simulink model "Clutch_Pedal"  (R2020b)
settings: Solver=VariableStepAuto  StartTime=0.0  StopTime=10.0  RelTol=1e-3
values from neighbouring files (symbols this model uses):
  be = 2.0    [clutch_parameters.sldd]
  bv = 1.0    [clutch_parameters.sldd]
  Ie = 1.0    [clutch_parameters.sldd]
  Iv = 5.0    [clutch_parameters.sldd]
  R = 1.0    [clutch_parameters.sldd]
  uk = 1.0    [clutch_parameters.sldd]
  us = 1.5    [clutch_parameters.sldd]
undefined symbols (not defined in the file or in its folder): sigbuilder_block
settings Model: DataDictionary=clutch_parameters.sldd  Creator=shivanshu shukla  LastModifiedBy=shivanshu shukla

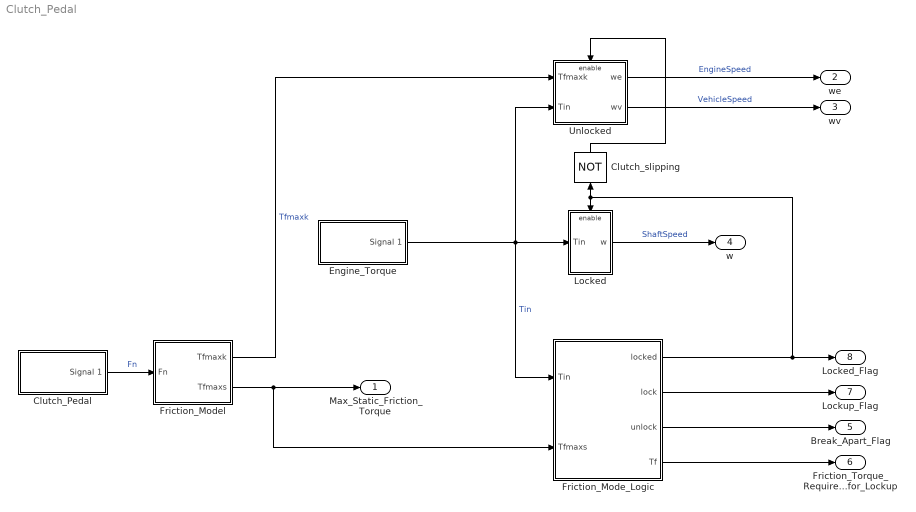
== system Clutch_Pedal ==
  Clutch_Pedal : Subsystem  Tag=STV Subsys  LoadFcn=sigbuilder_block('load');  StartFcn=sigbuilder_block('start');  StopFcn=sigbuilder_block('stop');  ClipboardFcn=sigbuilder_block('clipboard');  mask(Sigbuilder block){tuvar=[0:10]}
      mask help: Simulink:masks:SigbuilderBlock_MD
      mask init:
      | if ~strcmp(get_param(bdroot(gcbh),'SimulationStatus'),'stopped') tuvar = sigbuilder_block('maskInit'); end
      settings: CopyFcn=sigbuilder_block('copy');  DeleteFcn=sigbuilder_block('delete');  ModelCloseFcn=sigbuilder_block('modelClose');  PreSaveFcn=sigbuilder_block('preSave');  PauseFcn=sigbuilder_block('pause');  ContinueFcn=sigbuilder_block('continue');  NameChangeFcn=sigbuilder_block('namechange');  OpenFcn=sigbuilder_block('open',[437.6 153 550.4 359.25 ]);  CloseFcn=sigbuilder_block('close');
      mask Display: plot(0, 0, 100, 100,[2, 2, 32, 32, 2], [68, 8, 8, 68, 68],[32, 2], [38, 38], [32, 19, 2],[53, 60, 44], [32, 17, 17, 2],[16, 16, 31, 31]);txt = getActiveGroup(gcbh);text(2, 100, txt,'verticalAlignment', 'top');
  Clutch_slipping : Logic  Operator=NOT  IconShape=distinctive  AllPortsSameDT=off  OutDataTypeStr=boolean
  Engine_Torque : Subsystem  Tag=STV Subsys  LoadFcn=sigbuilder_block('load');  StartFcn=sigbuilder_block('start');  StopFcn=sigbuilder_block('stop');  ClipboardFcn=sigbuilder_block('clipboard');  mask(Sigbuilder block){tuvar=[0:10]}
      mask help: Simulink:masks:SigbuilderBlock_MD
      mask init:
      | if ~strcmp(get_param(bdroot(gcbh),'SimulationStatus'),'stopped') tuvar = sigbuilder_block('maskInit'); end
      settings: CopyFcn=sigbuilder_block('copy');  DeleteFcn=sigbuilder_block('delete');  ModelCloseFcn=sigbuilder_block('modelClose');  PreSaveFcn=sigbuilder_block('preSave');  PauseFcn=sigbuilder_block('pause');  ContinueFcn=sigbuilder_block('continue');  NameChangeFcn=sigbuilder_block('namechange');  OpenFcn=sigbuilder_block('open',[437.6 153 550.4 359.25 ]);  CloseFcn=sigbuilder_block('close');
      mask Display: plot(0, 0, 100, 100,[2, 2, 32, 32, 2], [68, 8, 8, 68, 68],[32, 2], [38, 38], [32, 19, 2],[53, 60, 44], [32, 17, 17, 2],[16, 16, 31, 31]);txt = getActiveGroup(gcbh);text(2, 100, txt,'verticalAlignment', 'top');
  Friction_Mode_Logic : Subsystem
  Friction_Model : Subsystem
  Locked : Subsystem
  Unlocked : Subsystem
  Max_Static_Friction_Torque : Outport
  we : Outport  Port=2
  wv : Outport  Port=3
  w : Outport  Port=4
  Break_Apart_Flag : Outport  Port=5
  Friction_Torque_Required_for_Lockup : Outport  Port=6
  Lockup_Flag : Outport  Port=7
  Locked_Flag : Outport  Port=8
  wires:
  Clutch_slipping/1 -> Unlocked/Enable
  Friction_Mode_Logic/1(locked) -> Locked_Flag/1, Clutch_slipping/1, Locked/Enable
  Friction_Model/1(Tfmaxk) -> Unlocked/1(Tfmaxk)  "Tfmaxk"
  Friction_Model/2(Tfmaxs) -> Max_Static_Friction_Torque/1, Friction_Mode_Logic/2(Tfmaxs)
  Engine_Torque/1(Signal 1) -> Friction_Mode_Logic/1(Tin), Locked/1(Tin), Unlocked/2(Tin)  "Tin"
  Clutch_Pedal/1(Signal 1) -> Friction_Model/1(Fn)  "Fn"
  Unlocked/1(we) -> we/1  "EngineSpeed"
  Unlocked/2(wv) -> wv/1  "VehicleSpeed"
  Locked/1(w) -> w/1  "ShaftSpeed"
  Friction_Mode_Logic/2(lock) -> Lockup_Flag/1
  Friction_Mode_Logic/3(unlock) -> Break_Apart_Flag/1
  Friction_Mode_Logic/4(Tf) -> Friction_Torque_Required_for_Lockup/1

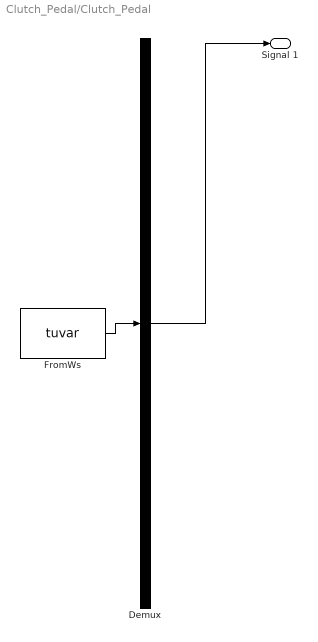
== system Clutch_Pedal/Clutch_Pedal ==
  Demux : Demux  Tag=STV Demux  Outputs=1
      settings: DisplayOption=none
  FromWs : FromWorkspace  Tag=STV FromWs  VariableName=tuvar
      SigBuilderData=|
      | common.afterFinalStr = 'Extrapolate'
      | common.sampleTime = 0
      | dataSet.timeRange = [0 10]
      | dataSet.name = 'Group 1'
      | sbobj.Groups.Name = 'Group 1'
      | sbobj.Groups.Signals.Name = 'Signal 1'
      | sbobj.Groups.Signals.XData = [0 1.98 3.96 4.98 6 7 7 10]
      | sbobj.Groups.Signals.YData = [0 1.6 1.6 1.6 0.83 -0.01 0 0]
  Signal 1 : Outport  Tag=STV Outport
  wires:
  Demux/1 -> Signal 1/1
  FromWs/1 -> Demux/1

== system Clutch_Pedal/Engine_Torque ==
  Demux : Demux  Tag=STV Demux  Outputs=1
      settings: DisplayOption=none
  FromWs : FromWorkspace  Tag=STV FromWs  VariableName=tuvar
      SigBuilderData=|
      | common.afterFinalStr = 'Extrapolate'
      | common.sampleTime = 0
      | dataSet.timeRange = [0 10]
      | dataSet.name = 'Group 1'
      | sbobj.Groups.Name = 'Group 1'
      | sbobj.Groups.Signals.Name = 'Signal 1'
      | sbobj.Groups.Signals.XData = [0 4 5.02 6 7 10]
      | sbobj.Groups.Signals.YData = [1.98 1.99 2 0.02 0 0]
  Signal 1 : Outport  Tag=STV Outport
  wires:
  Demux/1 -> Signal 1/1
  FromWs/1 -> Demux/1

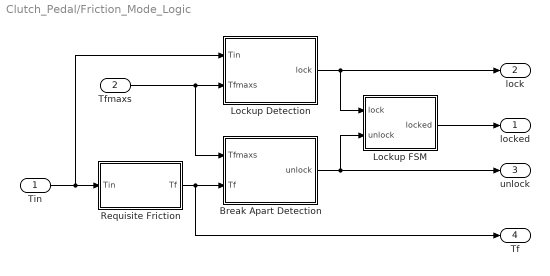
== system Clutch_Pedal/Friction_Mode_Logic ==
  Tin : Inport
  Tfmaxs : Inport  Port=2
  Break Apart Detection : Subsystem
  Lockup Detection : Subsystem
  Lockup FSM : Subsystem
  Requisite Friction : Subsystem
  locked : Outport  InitialOutput=0  VectorParamsAs1DForOutWhenUnconnected=off
  lock : Outport  Port=2  InitialOutput=0  VectorParamsAs1DForOutWhenUnconnected=off
  unlock : Outport  Port=3  InitialOutput=0  VectorParamsAs1DForOutWhenUnconnected=off
  Tf : Outport  Port=4  InitialOutput=0  VectorParamsAs1DForOutWhenUnconnected=off
  wires:
  Requisite Friction/1(Tf) -> Tf/1, Break Apart Detection/2(Tf)
  Break Apart Detection/1(unlock) -> unlock/1, Lockup FSM/2(unlock)
  Lockup FSM/1(locked) -> locked/1
  Tin/1 -> Lockup Detection/1(Tin), Requisite Friction/1(Tin)
  Lockup Detection/1(lock) -> lock/1, Lockup FSM/1(lock)
  Tfmaxs/1 -> Lockup Detection/2(Tfmaxs), Break Apart Detection/1(Tfmaxs)

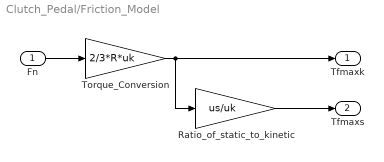
== system Clutch_Pedal/Friction_Model ==
  Fn : Inport
  Ratio_of_static_to_kinetic : Gain  Gain=us/uk  SaturateOnIntegerOverflow=on  OutDataTypeStr=Inherit: Same as input  ParamDataTypeStr=Inherit: Same as input
  Torque_Conversion : Gain  Gain=2/3*R*uk  SaturateOnIntegerOverflow=on  OutDataTypeStr=Inherit: Same as input  ParamDataTypeStr=Inherit: Same as input
  Tfmaxk : Outport  InitialOutput=0  VectorParamsAs1DForOutWhenUnconnected=off
  Tfmaxs : Outport  Port=2  InitialOutput=0  VectorParamsAs1DForOutWhenUnconnected=off
  wires:
  Torque_Conversion/1 -> Tfmaxk/1, Ratio_of_static_to_kinetic/1
  Ratio_of_static_to_kinetic/1 -> Tfmaxs/1
  Fn/1 -> Torque_Conversion/1

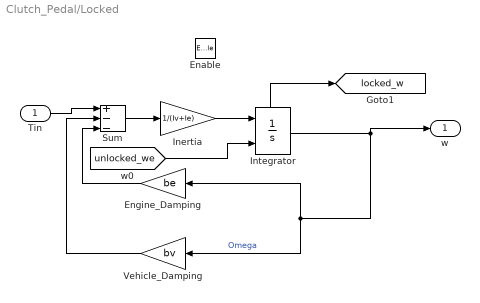
== system Clutch_Pedal/Locked ==
  Tin : Inport
  Enable : EnablePort  StatesWhenEnabling=reset
  Engine_Damping : Gain  Gain=be  SaturateOnIntegerOverflow=on  OutDataTypeStr=Inherit: Same as input  ParamDataTypeStr=Inherit: Same as input
  Inertia : Gain  Gain=1/(Iv+Ie)  SaturateOnIntegerOverflow=on  OutDataTypeStr=Inherit: Same as input  ParamDataTypeStr=Inherit: Same as input
  Integrator : Integrator  InitialConditionSource=external  ShowStatePort=on
  Sum : Sum  Inputs=+--  InputSameDT=on  SaturateOnIntegerOverflow=on  OutDataTypeStr=Inherit: Same as first input
  Vehicle_Damping : Gain  Gain=bv  SaturateOnIntegerOverflow=on  OutDataTypeStr=Inherit: Same as input  ParamDataTypeStr=Inherit: Same as input
  w : Outport  InitialOutput=0  VectorParamsAs1DForOutWhenUnconnected=off
  tag scope: locked_w=global
  wires:
  Engine_Damping/1 -> Sum/3
  Integrator/1 -> w/1, Engine_Damping/1, Vehicle_Damping/1  "Omega"
  Vehicle_Damping/1 -> Sum/2
  Tin/1 -> Sum/1
  Inertia/1 -> Integrator/1
  Sum/1 -> Inertia/1
  [unlocked_we] -> Integrator/2
  Integrator/State -> [locked_w]

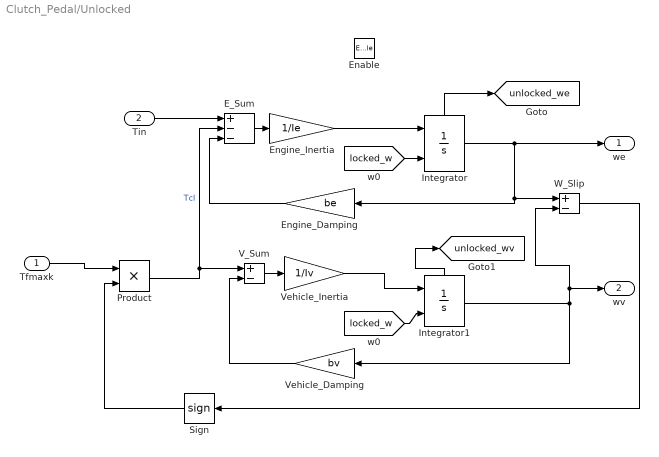
== system Clutch_Pedal/Unlocked ==
  Tfmaxk : Inport
  Tin : Inport  Port=2
  Enable : EnablePort
  E_Sum : Sum  Inputs=+--  InputSameDT=on  SaturateOnIntegerOverflow=on  OutDataTypeStr=Inherit: Same as first input
  Engine_Damping : Gain  Gain=be  SaturateOnIntegerOverflow=on  OutDataTypeStr=Inherit: Same as input  ParamDataTypeStr=Inherit: Same as input
  Engine_Inertia : Gain  Gain=1/Ie  SaturateOnIntegerOverflow=on  OutDataTypeStr=Inherit: Same as input  ParamDataTypeStr=Inherit: Same as input
  Integrator : Integrator  InitialConditionSource=external  ShowStatePort=on
  Integrator1 : Integrator  InitialConditionSource=external  ShowStatePort=on
  Product : Product
  Sign : Signum
  V_Sum : Sum  Inputs=+-  InputSameDT=on  SaturateOnIntegerOverflow=on  OutDataTypeStr=Inherit: Same as first input
  Vehicle_Damping : Gain  Gain=bv  SaturateOnIntegerOverflow=on  OutDataTypeStr=Inherit: Same as input  ParamDataTypeStr=Inherit: Same as input
  Vehicle_Inertia : Gain  Gain=1/Iv  SaturateOnIntegerOverflow=on  OutDataTypeStr=Inherit: Same as input  ParamDataTypeStr=Inherit: Same as input
  W_Slip : Sum  Inputs=+-  InputSameDT=on  SaturateOnIntegerOverflow=on  OutDataTypeStr=Inherit: Same as first input
  we : Outport  InitialOutput=0  VectorParamsAs1DForOutWhenUnconnected=off
  wv : Outport  Port=2  InitialOutput=0  VectorParamsAs1DForOutWhenUnconnected=off
  tag scope: unlocked_we=global, unlocked_wv=global
  wires:
  Vehicle_Damping/1 -> V_Sum/2
  Product/1 -> V_Sum/1, E_Sum/2  "Tcl"
  Vehicle_Inertia/1 -> Integrator1/1
  Tfmaxk/1 -> Product/1
  Integrator/1 -> we/1, Engine_Damping/1, W_Slip/1
  V_Sum/1 -> Vehicle_Inertia/1
  Engine_Damping/1 -> E_Sum/3
  Tin/1 -> E_Sum/1
  Integrator1/1 -> W_Slip/2, wv/1, Vehicle_Damping/1
  W_Slip/1 -> Sign/1
  E_Sum/1 -> Engine_Inertia/1
  Engine_Inertia/1 -> Integrator/1
  Sign/1 -> Product/2
  [locked_w] -> Integrator/2
  Integrator/State -> [unlocked_we]
  Integrator1/State -> [unlocked_wv]
  [locked_w] -> Integrator1/2

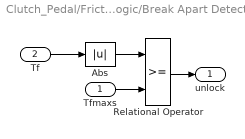
== system Clutch_Pedal/Friction_Mode_Logic/Break Apart Detection ==
  Tfmaxs : Inport
  Tf : Inport  Port=2
  Abs : Abs  SaturateOnIntegerOverflow=on
  Relational Operator : RelationalOperator  OutDataTypeStr=boolean  RndMeth=Nearest  InputSameDT=on
  unlock : Outport  InitialOutput=0  VectorParamsAs1DForOutWhenUnconnected=off
  wires:
  Tf/1 -> Abs/1
  Relational Operator/1 -> unlock/1
  Abs/1 -> Relational Operator/1
  Tfmaxs/1 -> Relational Operator/2

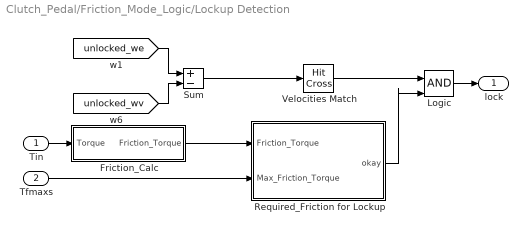
== system Clutch_Pedal/Friction_Mode_Logic/Lockup Detection ==
  Tin : Inport
  Tfmaxs : Inport  Port=2
  Friction_Calc : Subsystem
  Logic : Logic  IconShape=distinctive  OutDataTypeStr=boolean
  Required_Friction for Lockup : Subsystem
  Sum : Sum  Inputs=+-  InputSameDT=on  SaturateOnIntegerOverflow=on  OutDataTypeStr=Inherit: Same as first input
  Velocities Match : HitCross
  lock : Outport  InitialOutput=0  VectorParamsAs1DForOutWhenUnconnected=off
  wires:
  Tfmaxs/1 -> Required_Friction for Lockup/2(Max_Friction_Torque)
  Velocities Match/1 -> Logic/1
  Logic/1 -> lock/1
  Required_Friction for Lockup/1(okay) -> Logic/2
  [unlocked_we] -> Sum/1
  [unlocked_wv] -> Sum/2
  Sum/1 -> Velocities Match/1
  Tin/1 -> Friction_Calc/1(Torque)
  Friction_Calc/1(Friction_Torque) -> Required_Friction for Lockup/1(Friction_Torque)

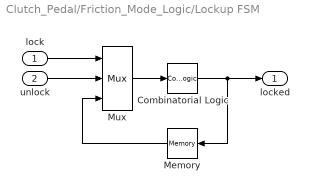
== system Clutch_Pedal/Friction_Mode_Logic/Lockup FSM ==
  lock : Inport
  unlock : Inport  Port=2
  Combinatorial Logic : CombinatorialLogic  TruthTable=[0;1;0;0;1;1;1;0]
  Memory : Memory
  Mux : Mux  Inputs=3
  locked : Outport  InitialOutput=0  VectorParamsAs1DForOutWhenUnconnected=off
  wires:
  Memory/1 -> Mux/3
  Combinatorial Logic/1 -> locked/1, Memory/1
  unlock/1 -> Mux/2
  lock/1 -> Mux/1
  Mux/1 -> Combinatorial Logic/1

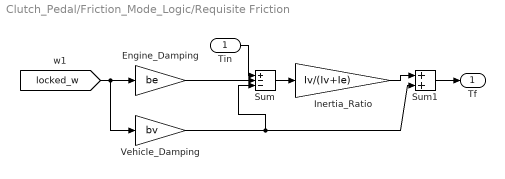
== system Clutch_Pedal/Friction_Mode_Logic/Requisite Friction ==
  Tin : Inport
  Engine_Damping : Gain  Gain=be  SaturateOnIntegerOverflow=on  OutDataTypeStr=Inherit: Same as input  ParamDataTypeStr=Inherit: Same as input
  Inertia_Ratio : Gain  Gain=Iv/(Iv+Ie)  SaturateOnIntegerOverflow=on  OutDataTypeStr=Inherit: Same as input  ParamDataTypeStr=Inherit: Same as input
  Sum : Sum  Inputs=+--  InputSameDT=on  SaturateOnIntegerOverflow=on  OutDataTypeStr=Inherit: Same as first input
  Sum1 : Sum  InputSameDT=on  SaturateOnIntegerOverflow=on  OutDataTypeStr=Inherit: Same as first input
  Vehicle_Damping : Gain  Gain=bv  SaturateOnIntegerOverflow=on  OutDataTypeStr=Inherit: Same as input  ParamDataTypeStr=Inherit: Same as input
  Tf : Outport  InitialOutput=0  VectorParamsAs1DForOutWhenUnconnected=off
  wires:
  [locked_w] -> Vehicle_Damping/1, Engine_Damping/1
  Engine_Damping/1 -> Sum/2
  Vehicle_Damping/1 -> Sum/3, Sum1/2
  Sum/1 -> Inertia_Ratio/1
  Tin/1 -> Sum/1
  Inertia_Ratio/1 -> Sum1/1
  Sum1/1 -> Tf/1

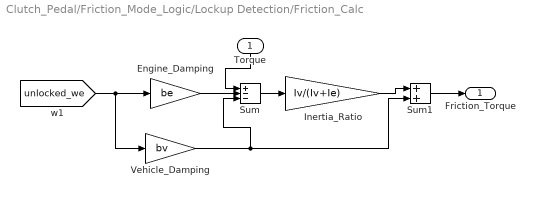
== system Clutch_Pedal/Friction_Mode_Logic/Lockup Detection/Friction_Calc ==
  Torque : Inport
  Engine_Damping : Gain  Gain=be  SaturateOnIntegerOverflow=on  OutDataTypeStr=Inherit: Same as input  ParamDataTypeStr=Inherit: Same as input
  Inertia_Ratio : Gain  Gain=Iv/(Iv+Ie)  SaturateOnIntegerOverflow=on  OutDataTypeStr=Inherit: Same as input  ParamDataTypeStr=Inherit: Same as input
  Sum : Sum  Inputs=+--  InputSameDT=on  SaturateOnIntegerOverflow=on  OutDataTypeStr=Inherit: Same as first input
  Sum1 : Sum  InputSameDT=on  SaturateOnIntegerOverflow=on  OutDataTypeStr=Inherit: Same as first input
  Vehicle_Damping : Gain  Gain=bv  SaturateOnIntegerOverflow=on  OutDataTypeStr=Inherit: Same as input  ParamDataTypeStr=Inherit: Same as input
  Friction_Torque : Outport  InitialOutput=0  VectorParamsAs1DForOutWhenUnconnected=off
  wires:
  Torque/1 -> Sum/1
  Sum1/1 -> Friction_Torque/1
  Vehicle_Damping/1 -> Sum1/2, Sum/3
  Sum/1 -> Inertia_Ratio/1
  Inertia_Ratio/1 -> Sum1/1
  Engine_Damping/1 -> Sum/2
  [unlocked_we] -> Engine_Damping/1, Vehicle_Damping/1

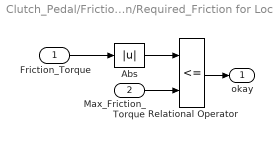
== system Clutch_Pedal/Friction_Mode_Logic/Lockup Detection/Required_Friction for Lockup ==
  Friction_Torque : Inport
  Max_Friction_Torque : Inport  Port=2
  Abs : Abs  SaturateOnIntegerOverflow=on
  Relational Operator : RelationalOperator  Operator=<=  OutDataTypeStr=boolean  RndMeth=Nearest  InputSameDT=on
  okay : Outport  InitialOutput=0  VectorParamsAs1DForOutWhenUnconnected=off
  wires:
  Friction_Torque/1 -> Abs/1
  Relational Operator/1 -> okay/1
  Abs/1 -> Relational Operator/1
  Max_Friction_Torque/1 -> Relational Operator/2
